simulink model "ADRC_DaoLiBai"  (R2018b)
settings: Solver=VariableStepAuto  StartTime=0.0  StopTime=30  RelTol=1e-3
settings Model: Creator=ILQMN  LastModifiedBy=ILQMN

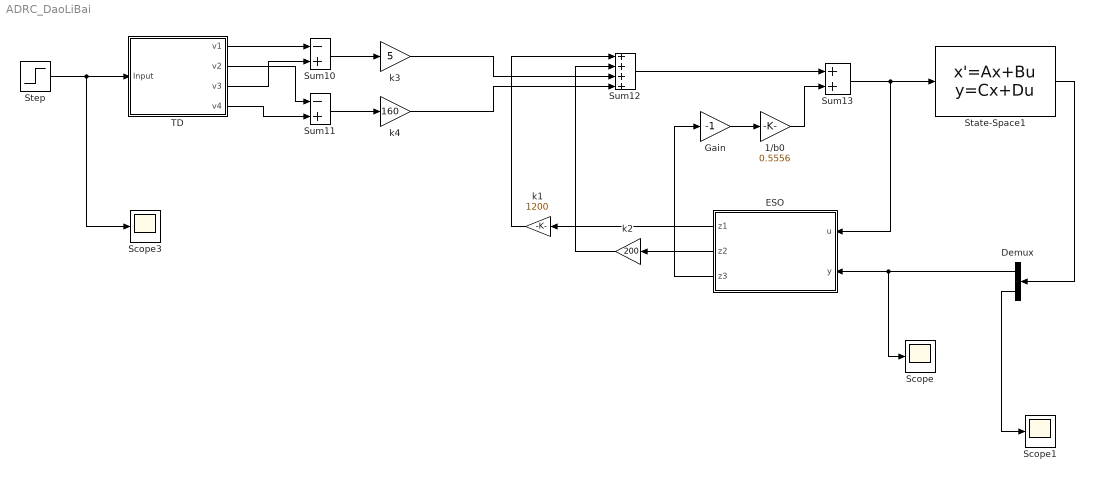
== system ADRC_DaoLiBai ==
  "1/b0 " : Gain  Gain=0.5556
  Demux : Demux  Outputs=2
  ESO : Subsystem
  Gain : Gain  Gain=-1
  Scope : Scope
  Scope1 : Scope
  Scope3 : Scope
  State-Space1 : StateSpace  A=[0 1 0 0;27.828 0 0 -0.2357;0 0 0 1;0.6393 0 0 -0.08832]  B=[0;2.6683;0;0.8832]  C=[1 0 0 0;0 0 1 0]  D=[0;0]  InitialCondition=[0;0;0;0]
  Step : Step  Time=0  SampleTime=0
  Sum10 : Sum  Inputs=-+
  Sum11 : Sum  Inputs=-+
  Sum12 : Sum  Inputs=++++
  Sum13 : Sum
  TD : Subsystem
  k1 : Gain  Gain=1200
  k2 : Gain  Gain=200
  k3 : Gain  Gain=5
  "k4 " : Gain  Gain=160
  wires:
  Step/1 -> Scope3/1, TD/1(Input)
  TD/1(v1) -> Sum10/1
  TD/3(v3) -> Sum10/2
  Sum10/1 -> k3/1
  TD/4(v4) -> Sum11/2
  TD/2("v2 ") -> Sum11/1
  Sum11/1 -> "k4 "/1
  k3/1 -> Sum12/3
  "k4 "/1 -> Sum12/4
  ESO/1(z1) -> k1/1
  ESO/2(z2) -> k2/1
  k1/1 -> Sum12/1
  k2/1 -> Sum12/2
  ESO/3(z3) -> Gain/1
  Gain/1 -> "1/b0 "/1
  Sum12/1 -> Sum13/1
  "1/b0 "/1 -> Sum13/2
  Sum13/1 -> State-Space1/1, ESO/1("u ")
  State-Space1/1 -> Demux/1
  Demux/1 -> Scope/1, ESO/2("y ")
  Demux/2 -> Scope1/1

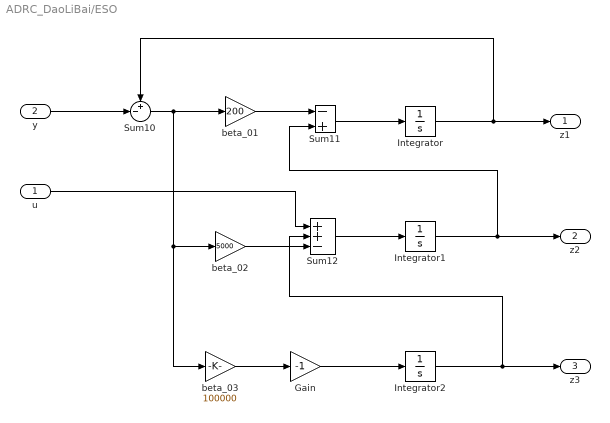
== system ADRC_DaoLiBai/ESO ==
  "u " : Inport
  "y " : Inport  Port=2
  Gain : Gain  Gain=-1
  Integrator : Integrator
  Integrator1 : Integrator
  Integrator2 : Integrator
  Sum10 : Sum  Inputs=+-|
  Sum11 : Sum  Inputs=-+
  Sum12 : Sum  Inputs=++-
  beta_01 : Gain  Gain=200
  beta_02 : Gain  Gain=5000
  beta_03 : Gain  Gain=100000
  z1 : Outport
  z2 : Outport  Port=2
  z3 : Outport  Port=3
  wires:
  beta_02/1 -> Sum12/3
  Gain/1 -> Integrator2/1
  Integrator1/1 -> Sum11/2, z2/1
  Integrator2/1 -> Sum12/2, z3/1
  Sum12/1 -> Integrator1/1
  "u "/1 -> Sum12/1
  beta_01/1 -> Sum11/1
  Sum10/1 -> beta_03/1, beta_02/1, beta_01/1
  Sum11/1 -> Integrator/1
  "y "/1 -> Sum10/2
  beta_03/1 -> Gain/1
  Integrator/1 -> z1/1, Sum10/1

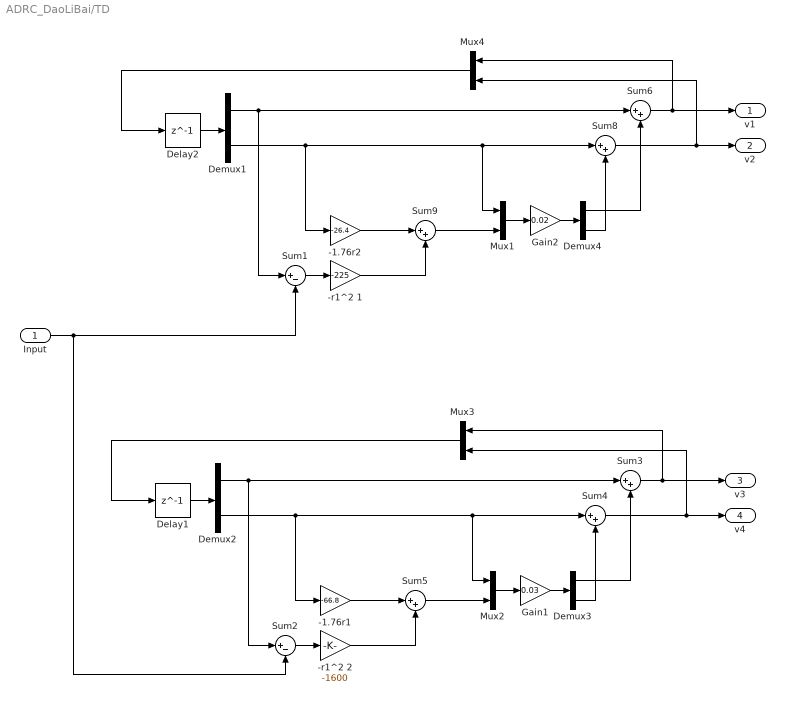
== system ADRC_DaoLiBai/TD ==
  Input : Inport
  -1.76r1 : Gain  Gain=-66.8
  -1.76r2 : Gain  Gain=-26.4
  -r1^2 1 : Gain  Gain=-225
  -r1^2 2 : Gain  Gain=-1600
  Delay1 : Delay  DelayLength=1
  Delay2 : Delay  DelayLength=1
  Demux{1..4} (4 alike) : Demux  Outputs=2
  Gain1 : Gain  Gain=0.03
  Gain2 : Gain  Gain=0.02
  Mux{1..4} (4 alike) : Mux  Inputs=2
  Sum1 : Sum  Inputs=|+-
  Sum2 : Sum  Inputs=|+-
  Sum{3..6,8..9} (6 alike) : Sum  Inputs=|++
  v1 : Outport
  "v2 " : Outport  Port=2
  v3 : Outport  Port=3
  v4 : Outport  Port=4
  wires:
  Demux1/2 -> -1.76r2/1, Mux1/1, Sum8/1
  Mux4/1 -> Delay2/1
  Sum9/1 -> Mux1/2
  Sum1/1 -> -r1^2 1/1
  Mux1/1 -> Gain2/1
  Demux4/1 -> Sum6/2
  Sum6/1 -> v1/1, Mux4/1
  Gain2/1 -> Demux4/1
  Demux4/2 -> Sum8/2
  Demux1/1 -> Sum6/1, Sum1/1
  -1.76r2/1 -> Sum9/1
  Delay2/1 -> Demux1/1
  -r1^2 1/1 -> Sum9/2
  Sum8/1 -> "v2 "/1, Mux4/2
  -1.76r1/1 -> Sum5/1
  Demux2/1 -> Sum3/1, Sum2/1
  Delay1/1 -> Demux2/1
  Sum4/1 -> v4/1, Mux3/2
  Mux3/1 -> Delay1/1
  Sum3/1 -> v3/1, Mux3/1
  Sum2/1 -> -r1^2 2/1
  Sum5/1 -> Mux2/2
  Mux2/1 -> Gain1/1
  Gain1/1 -> Demux3/1
  -r1^2 2/1 -> Sum5/2
  Demux2/2 -> -1.76r1/1, Mux2/1, Sum4/1
  Input/1 -> Sum1/2, Sum2/2
  Demux3/2 -> Sum4/2
  Demux3/1 -> Sum3/2
